simulink model "Factorial_usingForLoop"  (R2021a)
settings: Solver=VariableStepAuto  StartTime=0.0  StopTime=10.0  RelTol=1e-3
settings Model: Creator=NoteBook  LastModifiedBy=NoteBook

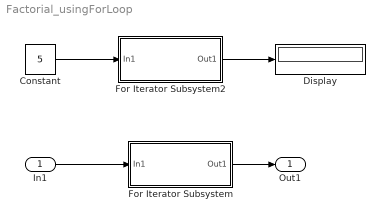
== system Factorial_usingForLoop ==
  In1 : Inport  OutDataTypeStr=uint16
  Constant : Constant  Value=5  OutDataTypeStr=uint16
  Display : Display
      settings: Format=decimal (Stored Integer)
  For Iterator Subsystem : Subsystem  TreatAsAtomicUnit=on
  For Iterator Subsystem2 : Subsystem  TreatAsAtomicUnit=on
  Out1 : Outport  OutDataTypeStr=uint16
  wires:
  For Iterator Subsystem2/1(Out1) -> Display/1
  For Iterator Subsystem/1(Out1) -> Out1/1
  In1/1 -> For Iterator Subsystem/1(In1)
  Constant/1 -> For Iterator Subsystem2/1(In1)

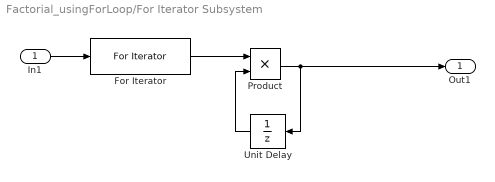
== system Factorial_usingForLoop/For Iterator Subsystem ==
  In1 : Inport
  For Iterator : ForIterator  IterationSource=external  IterationVariableDataType=uint16
  Product : Product  OutDataTypeStr=uint16
  Unit Delay : UnitDelay  InitialCondition=1  SampleTime=-1  HasFrameUpgradeWarning=on
  Out1 : Outport  OutDataTypeStr=uint16
  wires:
  For Iterator/1 -> Product/1
  Product/1 -> Unit Delay/1, Out1/1
  Unit Delay/1 -> Product/2
  In1/1 -> For Iterator/1

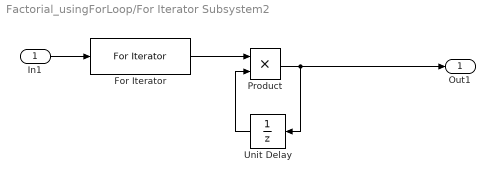
== system Factorial_usingForLoop/For Iterator Subsystem2 ==
  In1 : Inport
  For Iterator : ForIterator  ResetStates=reset  IterationSource=external  IterationVariableDataType=uint16
  Product : Product  OutDataTypeStr=uint16
  Unit Delay : UnitDelay  InitialCondition=1  SampleTime=-1  HasFrameUpgradeWarning=on
  Out1 : Outport  OutDataTypeStr=uint16
  wires:
  For Iterator/1 -> Product/1
  Product/1 -> Unit Delay/1, Out1/1
  Unit Delay/1 -> Product/2
  In1/1 -> For Iterator/1
